simulink model "PF_IE"  (R2018b)
settings: Solver=ode4  StartTime=0.0  StopTime=tfinal  FixedStep=1e-3  RelTol=1e-3
values from neighbouring files (symbols this model uses):
  hum_final = str2double(get(handles.humf,'string'))    [Humidity.m]    (also in settings.m = str2double(get(handles.rh_settings,'string')))
  temp_final = 0    [Humidity.m]    (also in settings.m = str2double(get(handles.temp_settings,'string')))
  wf_final = str2double(get(handles.wf_settings,'string'))    [settings.m]
libraries: simulink x2
settings Model: Creator=César  LastModifiedBy=César

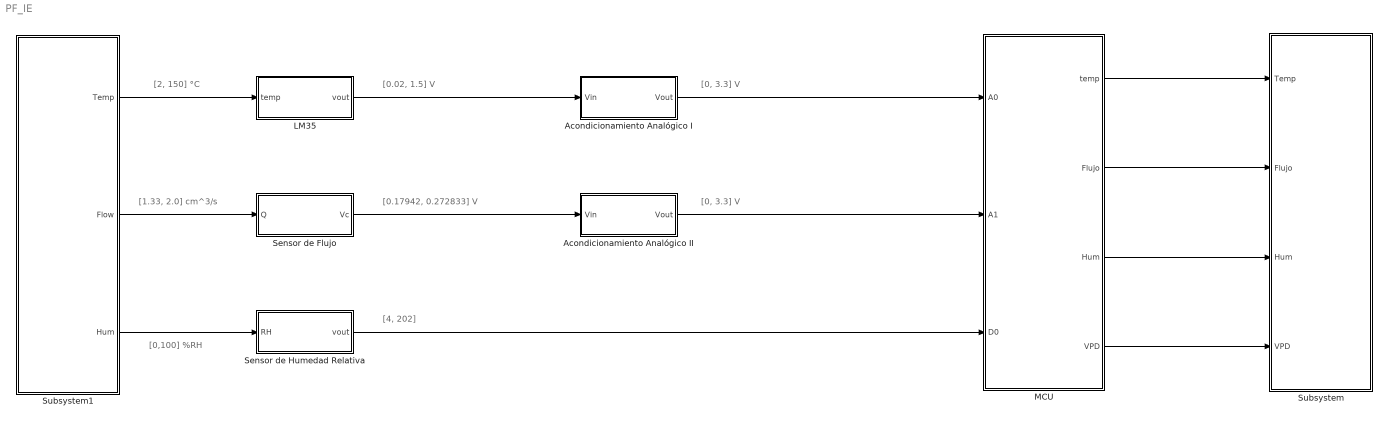
== system PF_IE ==
  note: [0, 3.3] V
  note: [0.02, 1.5] V
  note: [2, 150] °C
  note: [1.33, 2.0] cm^3/s
  note: [0.17942, 0.272833] V
  note: [0, 3.3] V
  note: [0,100] %RH
  note: [4, 202]
  Acondicionamiento Analógico I : Subsystem  Tag=LM35  Description=Temperature Sensor
  Acondicionamiento Analógico II : Subsystem  Tag=LM35  Description=Temperature Sensor
  LM35 : Subsystem  Tag=LM35  Description=Temperature Sensor
  MCU : Subsystem  Tag=LM35  Description=Temperature Sensor
  Sensor de Flujo : Subsystem  Tag=LM35  Description=Temperature Sensor
  Sensor de Humedad Relativa : Subsystem  Tag=LM35  Description=Temperature Sensor
  Subsystem : Subsystem
  Subsystem1 : Subsystem
  wires:
  Subsystem1/1(Temp) -> LM35/1("temp ")
  Acondicionamiento Analógico I/1("Vout ") -> MCU/1("A0 ")
  Sensor de Humedad Relativa/1("vout ") -> MCU/3("D0 ")
  Subsystem1/3(Hum) -> Sensor de Humedad Relativa/1("RH ")
  Subsystem1/2(Flow) -> Sensor de Flujo/1("Q ")
  Acondicionamiento Analógico II/1("Vout ") -> MCU/2("A1 ")
  Sensor de Flujo/1("Vc ") -> Acondicionamiento Analógico II/1("Vin ")
  LM35/1("vout ") -> Acondicionamiento Analógico I/1("Vin ")
  MCU/1("temp ") -> Subsystem/1(Temp)
  MCU/2(Flujo) -> Subsystem/2(Flujo)
  MCU/3("Hum ") -> Subsystem/3(Hum)
  MCU/4(VPD) -> Subsystem/4(VPD)

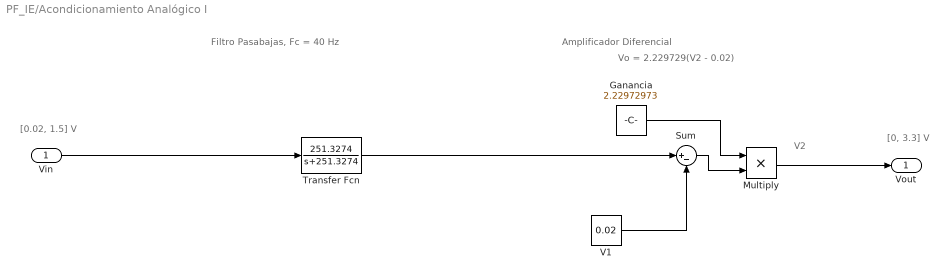
== system PF_IE/Acondicionamiento Analógico I ==
  note: Vo = 2.229729(V2 - 0.02)
  note: V2
  note: [0, 3.3] V
  note: Amplificador Diferencial
  note: [0.02, 1.5] V
  note: Filtro Pasabajas, Fc = 40 Hz
  "Vin " : Inport
  "Ganancia " : Constant  Value=2.22972973
  Multiply : Product
  Sum : Sum  Inputs=|+-
  Transfer Fcn : TransferFcn  Numerator=[251.3274]  Denominator=[1 251.3274]
  V1 : Constant  Value=0.02
  "Vout " : Outport
  wires:
  V1/1 -> Sum/2
  "Ganancia "/1 -> Multiply/1
  Sum/1 -> Multiply/2
  Multiply/1 -> "Vout "/1
  "Vin "/1 -> Transfer Fcn/1
  Transfer Fcn/1 -> Sum/1

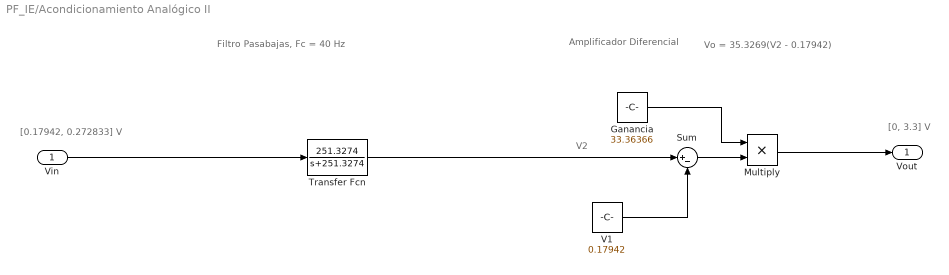
== system PF_IE/Acondicionamiento Analógico II ==
  note: Vo = 35.3269(V2 - 0.17942)
  note: V2
  note: [0, 3.3] V
  note: Amplificador Diferencial
  note: [0.17942, 0.272833] V
  note: Filtro Pasabajas, Fc = 40 Hz
  "Vin " : Inport
  "Ganancia " : Constant  Value=33.36366
  Multiply : Product
  Sum : Sum  Inputs=|+-
  Transfer Fcn : TransferFcn  Numerator=[251.3274]  Denominator=[1 251.3274]
  V1 : Constant  Value=0.17942
  "Vout " : Outport
  wires:
  Multiply/1 -> "Vout "/1
  V1/1 -> Sum/2
  "Ganancia "/1 -> Multiply/1
  Sum/1 -> Multiply/2
  "Vin "/1 -> Transfer Fcn/1
  Transfer Fcn/1 -> Sum/1

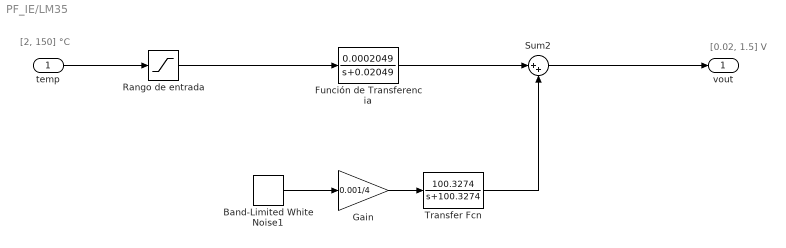
== system PF_IE/LM35 ==
  note: [0.02, 1.5] V
  note: [2, 150] °C
  "temp " : Inport
  Band-Limited White Noise1 : simulink/Sources/Band-Limited White Noise  Cov=[1]  Ts=1e-3  seed=[23341]
  Función de Transferencia : TransferFcn  Numerator=[0.0002049]  Denominator=[1 0.02049]
  Gain : Gain  Gain=0.001/4
  Rango de entrada : Saturate  UpperLimit=150  LowerLimit=2
  Sum2 : Sum  Inputs=|++
  Transfer Fcn : TransferFcn  Numerator=[100.3274]  Denominator=[1 100.3274]
  "vout " : Outport
  wires:
  Rango de entrada/1 -> Función de Transferencia/1
  Band-Limited White Noise1/1 -> Gain/1
  Función de Transferencia/1 -> Sum2/1
  "temp "/1 -> Rango de entrada/1
  Sum2/1 -> "vout "/1
  Gain/1 -> Transfer Fcn/1
  Transfer Fcn/1 -> Sum2/2

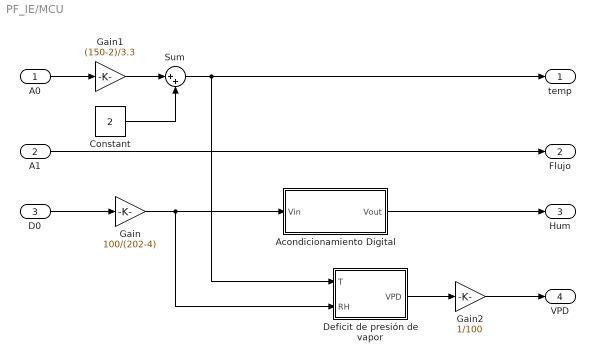
== system PF_IE/MCU ==
  "A0 " : Inport
  "A1 " : Inport  Port=2
  "D0 " : Inport  Port=3
  "Acondicionamiento Digital " : Subsystem  Tag=LM35  Description=Temperature Sensor
  Constant : Constant  Value=2
  Deficit de presión de vapor : MATLAB Function  TreatAsAtomicUnit=on
  Gain : Gain  Gain=100/(202-4)
  Gain1 : Gain  Gain=(150-2)/3.3
  Gain2 : Gain  Gain=1/100
  Sum : Sum  Inputs=|++
  "temp " : Outport
  Flujo : Outport  Port=2
  "Hum " : Outport  Port=3
  VPD : Outport  Port=4
  wires:
  Sum/1 -> "temp "/1, Deficit de presión de vapor/1(T)
  "Acondicionamiento Digital "/1("Vout ") -> "Hum "/1
  "A1 "/1 -> Flujo/1
  "D0 "/1 -> Gain/1
  Gain/1 -> Deficit de presión de vapor/2(RH), "Acondicionamiento Digital "/1("Vin ")
  "A0 "/1 -> Gain1/1
  Deficit de presión de vapor/1(VPD) -> Gain2/1
  Gain2/1 -> VPD/1
  Gain1/1 -> Sum/1
  Constant/1 -> Sum/2

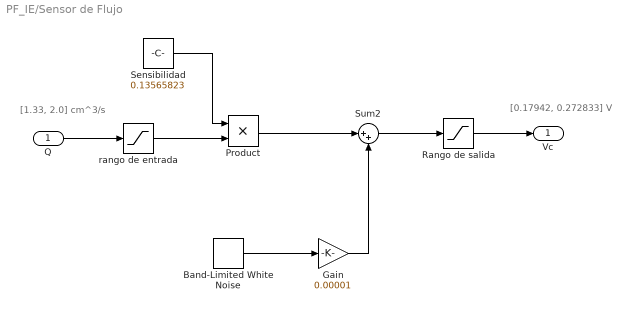
== system PF_IE/Sensor de Flujo ==
  note: [1.33, 2.0] cm^3/s
  note: [0.17942, 0.272833] V
  "Q " : Inport
  Band-Limited White Noise : simulink/Sources/Band-Limited White Noise  Cov=[0.01]  Ts=1e-3  seed=[23341]
  Gain : Gain  Gain=0.00001
  Product : Product
  Rango de salida : Saturate  UpperLimit=0.28  LowerLimit=0.16
  Sensibilidad : Constant  Value=0.13565823
  Sum2 : Sum  Inputs=|++
  rango de entrada : Saturate  UpperLimit=2.0  LowerLimit=1.32
  "Vc " : Outport
  wires:
  Sensibilidad/1 -> Product/1
  "Q "/1 -> rango de entrada/1
  rango de entrada/1 -> Product/2
  Sum2/1 -> Rango de salida/1
  Product/1 -> Sum2/1
  Gain/1 -> Sum2/2
  Band-Limited White Noise/1 -> Gain/1
  Rango de salida/1 -> "Vc "/1

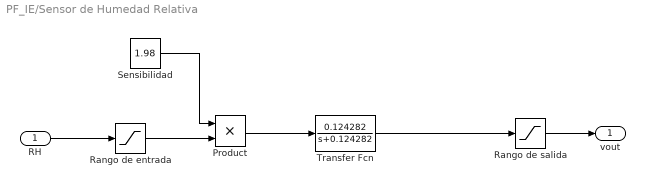
== system PF_IE/Sensor de Humedad Relativa ==
  "RH " : Inport
  Product : Product
  Rango de entrada : Saturate  UpperLimit=100  LowerLimit=0
  Rango de salida : Saturate  UpperLimit=255  LowerLimit=0
  Sensibilidad : Constant  Value=1.98
  Transfer Fcn : TransferFcn  Numerator=[0.124282]  Denominator=[1 0.124282]
  "vout " : Outport
  wires:
  Product/1 -> Transfer Fcn/1
  Sensibilidad/1 -> Product/1
  "RH "/1 -> Rango de entrada/1
  Rango de entrada/1 -> Product/2
  Rango de salida/1 -> "vout "/1
  Transfer Fcn/1 -> Rango de salida/1

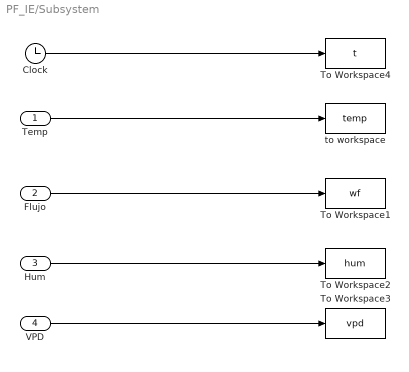
== system PF_IE/Subsystem ==
  Temp : Inport
  Flujo : Inport  Port=2
  Hum : Inport  Port=3
  VPD : Inport  Port=4
  Clock : Clock
  To Workspace1 : ToWorkspace  VariableName=wf  SampleTime=-1
  To Workspace2 : ToWorkspace  VariableName=hum  SampleTime=-1
  To Workspace3 : ToWorkspace  VariableName=vpd  SaveFormat=Timeseries  SampleTime=-1
  To Workspace4 : ToWorkspace  VariableName=t  SampleTime=-1
  to workspace : ToWorkspace  VariableName=temp  SampleTime=-1
  wires:
  Temp/1 -> to workspace/1
  Flujo/1 -> To Workspace1/1
  Hum/1 -> To Workspace2/1
  VPD/1 -> To Workspace3/1
  Clock/1 -> To Workspace4/1

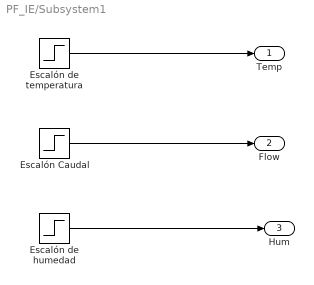
== system PF_IE/Subsystem1 ==
  Escalón Caudal : Step  After=wf_final  SampleTime=0
  "Escalón de humedad " : Step  After=hum_final  SampleTime=0
  Escalón de temperatura : Step  Time=2  After=temp_final  SampleTime=0
  Temp : Outport
  Flow : Outport  Port=2
  Hum : Outport  Port=3
  wires:
  Escalón de temperatura/1 -> Temp/1
  Escalón Caudal/1 -> Flow/1
  "Escalón de humedad "/1 -> Hum/1

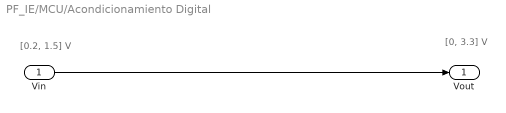
== system PF_IE/MCU/Acondicionamiento Digital  ==
  note: [0, 3.3] V
  note: [0.2, 1.5] V
  "Vin " : Inport
  "Vout " : Outport
  wires:
  "Vin "/1 -> "Vout "/1

== matlab function PF_IE/MCU/Deficit de presión de vapor ==
  data: T input; VPD output; RH input
function VPD = fcn(T,RH)

VPD = exp(6.41+(0.0727*T)-(3e-4*(T^2))+(1.18e-6*(T^3))-(3.86e-9*(T^4)))*(1-(RH/100));
